simulink model "corr_test"  (Simulink 7.3)
settings: Solver=ode45  StartTime=0.0  StopTime=10000  RelTol=1e-3
libraries: xbsIndex_r4 x689, dali_library x32, dspsigops x2, xps_library x2, simulink x1, casper_library x1
(part 1 of 7)
settings Model: Creator=rprimian  LastModifiedBy=rprimian

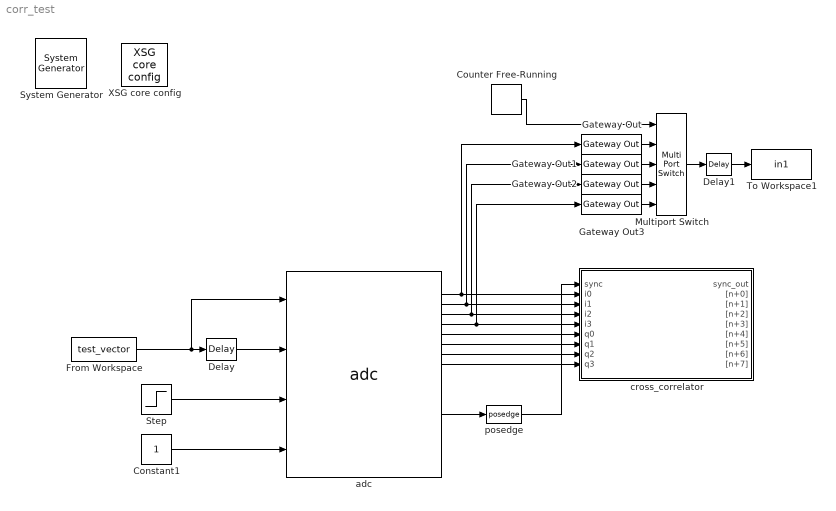
== system corr_test ==
  " System Generator" : xbsIndex_r4/ System Generator  Tag=genX  SystemSampleTime=-1  xilinxfamily=Virtex6  part=xc6vsx315t  speed=-3  package=ff1156  synthesis_tool=XST  clock_wrapper=Clock Enables  directory=./netlist  testbench=off  simulink_period=1  sysclk_period=10  dcm_input_clock_period=10  incr_netlist=off  trim_vbits=Everywhere in SubSystem  dbl_ovrd=According to Block Masks  core_generation=According to Block Masks  run_coregen=off  deprecated_control=off  eval_field=0  block_type=sysgen
      settings: block_version=11.3
  Constant1 : Constant  OutDataType=fixdt(1, 16)  OutScaling=2^0
  Counter Free-Running : simulink/Sources/Counter Free-Running  SystemSampleTime=-1  NumBits=2  tsamp=0.25
  Delay : dspsigops/Delay  dly_unit=Samples  delay=4  ic_detail=off  dif_ic_for_ch=off  dif_ic_for_dly=off  ic=0  reset_popup=None
  Delay1 : dspsigops/Delay  dly_unit=Samples  delay=4+7  ic_detail=off  dif_ic_for_ch=off  dif_ic_for_dly=off  ic=0  reset_popup=None
  From Workspace : FromWorkspace  VariableName=test_vector  SampleTime=0.25  Interpolate=off  OutputAfterFinalValue=Setting to zero
  Gateway Out{,1..3} (4 alike) : xbsIndex_r4/Gateway Out  hdl_port=on  timing_constraint=None  locs_specified=off  LOCs={}  block_type=gatewayout
      settings: infoedit="Gateway out block.  Converts Xilinx fixed point inputs into ouputs of type Simulink integer, double, or fixed point.<br><br>Hardware notes:  In hardware these blocks become top level output ports or are discarded, depending on how they are configured."  block_version=11.3
  Multiport Switch : MultiPortSwitch  Inputs=4  zeroidx=on  OutDataType=fixdt(1, 16)  OutScaling=2^0
  Step : Step  SampleTime=0
  To Workspace1 : ToWorkspace  VariableName=in1  SampleTime=-1  SaveFormat=Array
      settings: MaxDataPoints=40000
  XSG core config : xps_library/XSG core config  Tag=xps:xsg  SystemSampleTime=-1  hw_sys=ROACH:sx95t  ibob_linux=off  clk_src=adc0_clk  iBOB_clk_src=sys_clk  BEE2_ctrl_clk_src=sys_clk  BEE2_usr_clk_src=sys_clk  ROACH_clk_src=adc0_clk  CORR_clk_src=sys_clk  gpio_clk_io_group=iBOB:sma  gpio_clk_bit_index=0  clk_rate=200  sample_period=1  synthesis_tool=XST  mpc_type=powerpc440_ext
  adc : xps_library/adc  Tag=xps:adc  SystemSampleTime=-1  adc_brd=adc0  adc_clk_rate=800  adc_interleave=off  sample_period=1
  cross_correlator : Subsystem  AncestorBlock=dali_library/cross_correlator  mask(cross_correlator){total_lags=5, n_inputs=2, input_bit_width=8, input_bin_pt=7, specify_data_type=off, output_bit_width=16, output_bin_pt=14, quantization=Truncate, overflow=Wrap, specify_mult=off, mult_spec=Behavioral, specify_add=off, add_spec=Fabric, mult_delay=3, add_delay=2}
      mask prompts: total_lags "Total Lags Centered at Zero: (2^?)"; n_inputs "Number of Simultaneous Inputs: (2^?)"; input_bit_width "Input Bit Width:"; input_bin_pt "Input Binary Point:"; specify_data_type "Specify output data type"; output_bit_width "Output Bit Width:"; output_bin_pt "Output Binary Point:"; quantization "Quantization Behavior:"; overflow "Overflow Behavior"; specify_mult "Specify multiplier use (behavioural HDL if not specified)"; mult_spec "Multiplier specification:"; specify_add "Specify adder use (behavioural HDL if not specified)"; add_spec "Adder specification:"; mult_delay "Mult Latency:"; add_delay "Add Latency:"
      mask help: This time-domain cross correlator accepts two real time-series and outputs the cross-correlation function for the given set of lags. The output is accumulated so that for every two input samples there is exactly one output sample.
      mask init:
      | cross_correlator_init(gcb,...
      |     'total_lags', total_lags,...
      |     'n_inputs', n_inputs,...
      |     'input_bit_width', input_bit_width,...
      |     'input_bin_pt', input_bin_pt,...
      |     'specify_data_type', specify_data_type,...
      |     'output_bit_width', output_bit_width,...
      |     'output_bin_pt', output_bin_pt,...
      |     'quantization', quantization,...
      |     'overflow', overflow,...
      |     'specify_mult', specify_mult,...
      |     'mult_spec', mult_spec,...
      |     'specify_add', specify_add,...
      |     'add_spec', add_spec,...
      |     'mult_delay', mult_delay,...
      |     'add_delay', add_delay);
      settings: AttributesFormatString=|
      | 32 lags, Demux: 4,
      | 8_7=>16_14, Truncate, Wrap
      |  Mult: Behavioral, Add: Fabric
      mask StyleString: edit,edit,edit,edit,checkbox,edit,edit,popup(Truncate|Round (unbiased: +/- Inf)|Round (unbiased: Even Values)),popup(Wrap|Saturate|Error),checkbox,popup(Behavioral|Core|Embedded),checkbox,popup(Fabric|DSP48),edit,edit
      mask CallbackString:
      | ||||specify_data_type = get_param(gcb,'specify_data_type');
      | visibs = get_param(gcb, 'MaskVisibilities');
      | if( strcmp(specify_data_type,'off')),
      |     visibs{6} = 'off';
      |     visibs{7} = 'off';
      |     visibs{8} = 'off';
      |     visibs{9} = 'off';
      | else
      |     visibs{6} = 'on';
      |     visibs{7} = 'on';
      |     visibs{8} = 'on';
      |     visibs{9} = 'on';
      | end
      | set_param(gcb, 'MaskVisibilities', visibs);
      | |||||specify_mult = get_param(gcb,'specify_mult');
      | visibs = get_param(gcb, 'MaskVisibilities');
      | if( strcmp(specify_mult,'off')),
      |     visibs{11} = 'off';
      | else
      |     visibs{11} = 'on';
      | end
      | set_param(gcb, 'MaskVisibilities', visibs);
      | ||specify_add = get_param(gcb,'specify_add');
      | visibs = get_param(gcb, 'MaskVisibilities');
      | if( strcmp(specify_add,'off')),
      |     visibs{13} = 'off';
      | else
      |     visibs{13} = 'on';
      | end
      | set_param(gcb, 'MaskVisibilities', visibs);
      | |||
  posedge : casper_library/Misc/posedge  Tag=Rising Edge Detector  SystemSampleTime=-1
  wires:
  From Workspace/1 -> Delay/1, adc/1
  adc/1 -> Gateway Out/1, cross_correlator/2(i0)
  adc/2 -> Gateway Out1/1, cross_correlator/3(i1)
  adc/3 -> Gateway Out2/1, cross_correlator/4(i2)
  adc/4 -> Gateway Out3/1, cross_correlator/5(i3)
  adc/5 -> cross_correlator/6(q0)
  adc/6 -> cross_correlator/7(q1)
  adc/7 -> cross_correlator/8(q2)
  adc/8 -> cross_correlator/9(q3)
  Delay/1 -> adc/2
  Step/1 -> adc/3
  Constant1/1 -> adc/4
  Counter Free-Running/1 -> Multiport Switch/1
  Gateway Out/1 -> Multiport Switch/2
  Gateway Out1/1 -> Multiport Switch/3
  Gateway Out2/1 -> Multiport Switch/4
  Gateway Out3/1 -> Multiport Switch/5
  Multiport Switch/1 -> Delay1/1
  Delay1/1 -> To Workspace1/1
  adc/13 -> posedge/1
  posedge/1 -> cross_correlator/1(sync)
